simulink subsystem "User_Interface_Dashboard"  (R2024b)
settings: Solver=VariableStepAuto  StartTime=0.0  StopTime=10.0  RelTol=1e-3
undefined symbols (not defined in the file): NrLEDStrips, operatingMode, ts1ms, ts500us
libraries: SEPIC_utilities x6, simulink x1
settings Model: Creator=vlenzi  LastModifiedBy=vlenzi

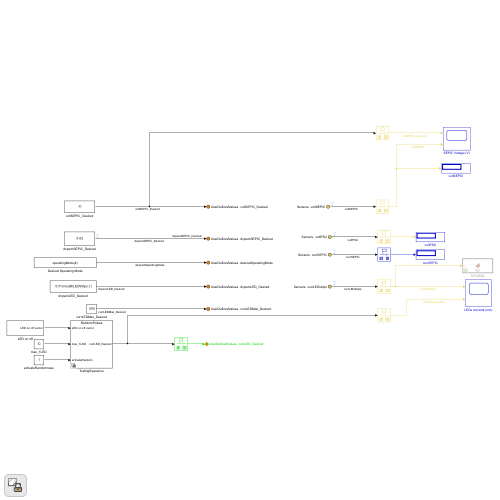
[thumbnail: Simulink's stored preview of the top-level diagram]
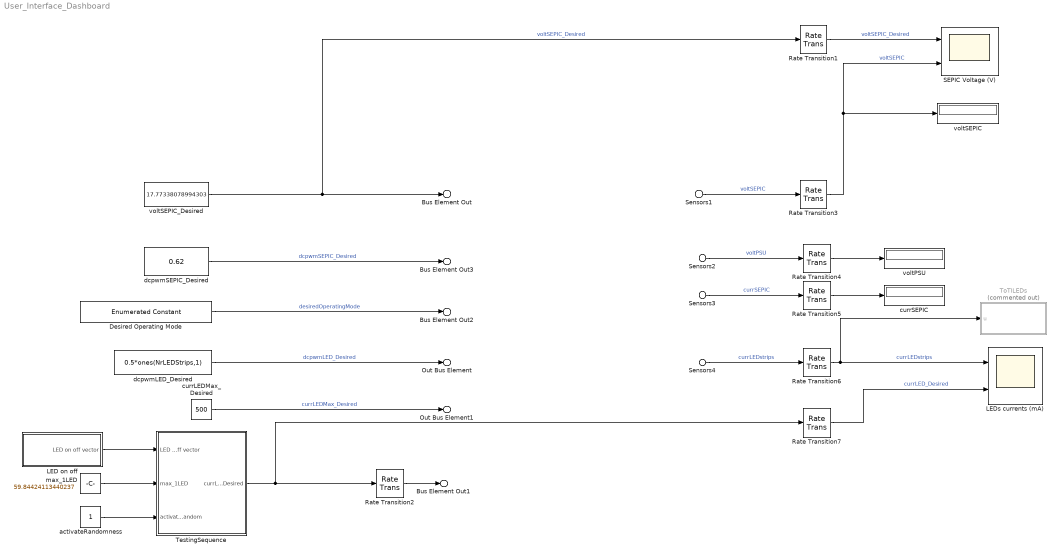
== system User_Interface_Dashboard ==
  Sensors1 : Inport  PortName=Sensors  Element=voltSEPIC
  Sensors3 : Inport  PortName=Sensors  Element=currSEPIC
  Sensors4 : Inport  PortName=Sensors  Element=currLEDstrips
  Sensors2 : Inport  PortName=Sensors  Element=voltPSU
  Desired Operating Mode : simulink/Sources/Enumerated Constant  OutDataTypeStr=Enum: operatingMode  Value=operatingMode(4)  SampleTime=-1
  LED on off : Subsystem
  LEDs currents (mA) : Scope  NumInputPorts=2
  Rate Transition{1,3..7} (6 alike) : RateTransition  Deterministic=off  OutPortSampleTime=ts10ms
  Rate Transition2 : RateTransition  Deterministic=off
  SEPIC Voltage (V) : Scope  NumInputPorts=2
  TestingSequence : Subsystem  Variant=on  VariantControlMode=label  VariantControl=Choice  LabelModeActiveChoice=Choice_1
  ToTILEDs : MATLAB Function  Commented=on  TreatAsAtomicUnit=on
  activateRandomness : Constant  OutDataTypeStr=single  SampleTime=-1
  currLEDMax_Desired : Constant  Value=500  OutDataTypeStr=single  SampleTime=-1
  currSEPIC : Display
  dcpwmLED_Desired : Constant  Value=0.5*ones(NrLEDStrips,1)  OutDataTypeStr=single  SampleTime=-1
  dcpwmSEPIC_Desired : Constant  Value=0.62  OutDataTypeStr=single  SampleTime=-1
  max_1LED : Constant  Value=59.84424113440237  OutDataTypeStr=single  SampleTime=-1
  voltPSU : Display
  voltSEPIC : Display
  voltSEPIC_Desired : Constant  Value=17.77338078994303  OutDataTypeStr=single  SampleTime=-1
  Bus Element Out1 : Outport  PortName=UserDefinedValues  Element=currLED_Desired
  Out Bus Element1 : Outport  PortName=UserDefinedValues  Element=currLEDMax_Desired
  Bus Element Out3 : Outport  PortName=UserDefinedValues  Element=dcpwmSEPIC_Desired
  Out Bus Element : Outport  PortName=UserDefinedValues  Element=dcpwmLED_Desired
  Bus Element Out2 : Outport  PortName=UserDefinedValues  Element=desiredOperatingMode
  Bus Element Out : Outport  PortName=UserDefinedValues  Element=voltSEPIC_Desired
  wires:
  voltSEPIC_Desired/1 -> Rate Transition1/1, Bus Element Out/1  "voltSEPIC_Desired"
  Desired Operating Mode/1 -> Bus Element Out2/1  "desiredOperatingMode"
  Sensors1/1 -> Rate Transition3/1  "voltSEPIC"
  Sensors2/1 -> Rate Transition4/1  "voltPSU"
  Sensors3/1 -> Rate Transition5/1  "currSEPIC"
  Sensors4/1 -> Rate Transition6/1  "currLEDstrips"
  dcpwmSEPIC_Desired/1 -> Bus Element Out3/1  "dcpwmSEPIC_Desired"
  dcpwmLED_Desired/1 -> Out Bus Element/1  "dcpwmLED_Desired"
  Rate Transition6/1 -> ToTILEDs/1(u), LEDs currents (mA)/1  "currLEDstrips"
  currLEDMax_Desired/1 -> Out Bus Element1/1  "currLEDMax_Desired"
  Rate Transition3/1 -> SEPIC Voltage (V)/2, voltSEPIC/1  "voltSEPIC"
  Rate Transition4/1 -> voltPSU/1
  Rate Transition5/1 -> currSEPIC/1
  Rate Transition1/1 -> SEPIC Voltage (V)/1  "voltSEPIC_Desired"
  TestingSequence/1(currLED_Desired) -> Rate Transition7/1, Rate Transition2/1
  Rate Transition7/1 -> LEDs currents (mA)/2  "currLED_Desired"
  max_1LED/1 -> TestingSequence/2(max_1LED)
  LED on off/1(LED on off vector) -> TestingSequence/1(LED on off vector)
  activateRandomness/1 -> TestingSequence/3(activateRandom)
  Rate Transition2/1 -> Bus Element Out1/1

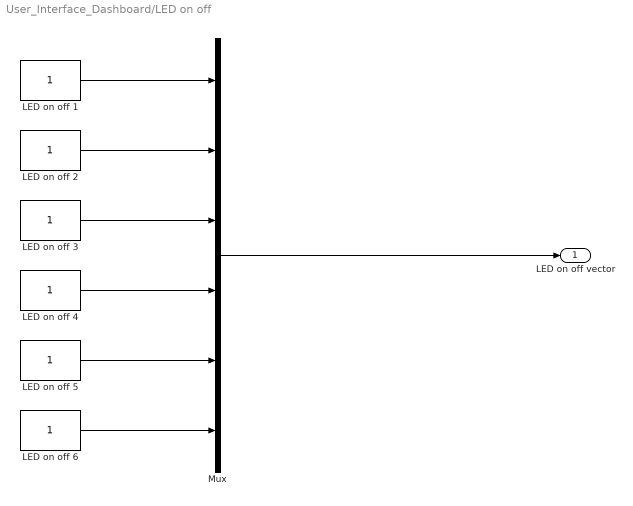
== system User_Interface_Dashboard/LED on off ==
  LED on off {1..6} (6 alike) : Constant  OutDataTypeStr=single  SampleTime=-1
  Mux : Mux  Inputs=6
  LED on off vector : Outport
  wires:
  LED on off 3/1 -> Mux/3
  LED on off 5/1 -> Mux/5
  LED on off 1/1 -> Mux/1
  LED on off 4/1 -> Mux/4
  LED on off 2/1 -> Mux/2
  LED on off 6/1 -> Mux/6
  Mux/1 -> LED on off vector/1

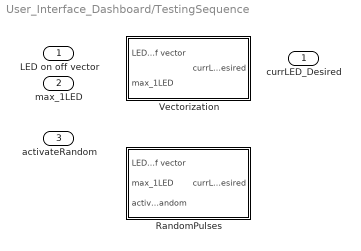
== system User_Interface_Dashboard/TestingSequence ==
  LED on off vector : Inport
  max_1LED : Inport  Port=2
  activateRandom : Inport  Port=3
  RandomPulses : Subsystem  VariantControl=Choice_1
  Vectorization : Subsystem  VariantControl=Choice
  currLED_Desired : Outport

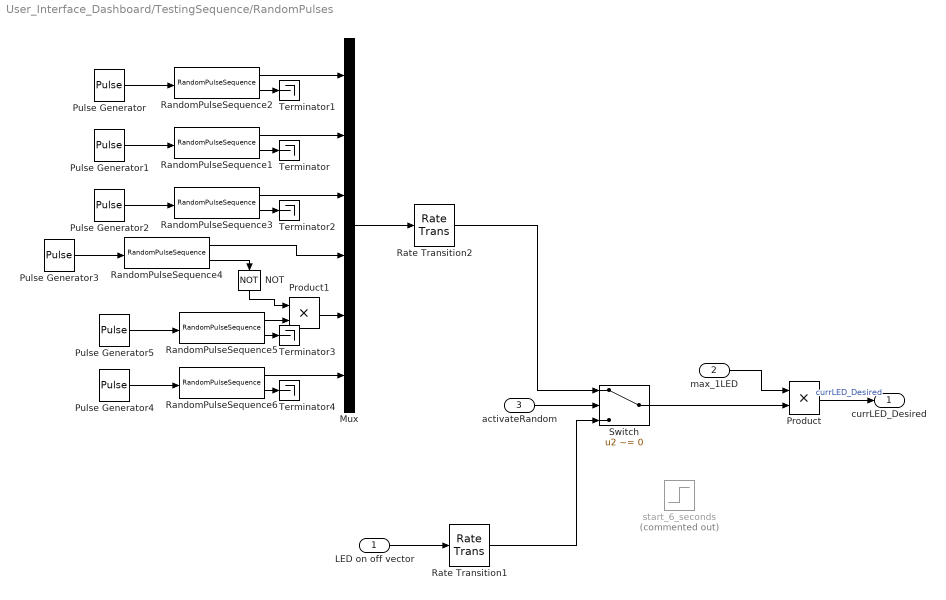
== system User_Interface_Dashboard/TestingSequence/RandomPulses ==
  LED on off vector : Inport
  max_1LED : Inport  Port=2
  activateRandom : Inport  Port=3
  Mux : Mux  Inputs=6
  NOT : Logic  Operator=NOT  AllPortsSameDT=off  OutDataTypeStr=boolean
  Product : Product  OutDataTypeStr=single
  Product1 : Product
  Pulse Generator : DiscretePulseGenerator  Period=2*(1/ts500us)  PulseWidth=1*(1/ts500us)  SampleTime=ts500us
  Pulse Generator1 : DiscretePulseGenerator  Period=2*(1/ts500us)  PulseWidth=1*(1/ts500us)  PhaseDelay=1*400  SampleTime=ts500us
  Pulse Generator2 : DiscretePulseGenerator  Period=2*(1/ts500us)  PulseWidth=1*(1/ts500us)  PhaseDelay=2*400  SampleTime=ts500us
  Pulse Generator3 : DiscretePulseGenerator  Period=2*(1/ts500us)  PulseWidth=1*(1/ts500us)  PhaseDelay=3*400  SampleTime=ts500us
  Pulse Generator4 : DiscretePulseGenerator  Period=2*(1/ts500us)  PulseWidth=1*(1/ts500us)  PhaseDelay=5*400  SampleTime=ts500us
  Pulse Generator5 : DiscretePulseGenerator  Period=2*(1/ts500us)  PulseWidth=1*(1/ts500us)  PhaseDelay=4*400  SampleTime=ts500us
  RandomPulseSequence1 : SEPIC_utilities/RandomPulseSequence  seed=2  sampleTime=4
  RandomPulseSequence2 : SEPIC_utilities/RandomPulseSequence  seed=1  sampleTime=4
  RandomPulseSequence3 : SEPIC_utilities/RandomPulseSequence  seed=3  sampleTime=4
  RandomPulseSequence4 : SEPIC_utilities/RandomPulseSequence  seed=4  sampleTime=4
  RandomPulseSequence5 : SEPIC_utilities/RandomPulseSequence  seed=5  sampleTime=4
  RandomPulseSequence6 : SEPIC_utilities/RandomPulseSequence  seed=6  sampleTime=4
  Rate Transition1 : RateTransition  Deterministic=off
  Rate Transition2 : RateTransition  Deterministic=off
  Switch : Switch  Criteria=u2 ~= 0  SaturateOnIntegerOverflow=off  InputSameDT=off
  Terminator{,1..4} (5 alike) : Terminator
  start_6_seconds : Step  Commented=on  Time=6  SampleTime=ts1ms
  currLED_Desired : Outport
  wires:
  Rate Transition1/1 -> Switch/3
  Rate Transition2/1 -> Switch/1
  LED on off vector/1 -> Rate Transition1/1
  Switch/1 -> Product/2
  activateRandom/1 -> Switch/2
  max_1LED/1 -> Product/1
  Product/1 -> currLED_Desired/1  "currLED_Desired"
  RandomPulseSequence3/2 -> Terminator2/1
  RandomPulseSequence2/1 -> Mux/1
  RandomPulseSequence5/1 -> Product1/2
  Pulse Generator4/1 -> RandomPulseSequence6/1
  Mux/1 -> Rate Transition2/1
  Pulse Generator5/1 -> RandomPulseSequence5/1
  Pulse Generator1/1 -> RandomPulseSequence1/1
  NOT/1 -> Product1/1
  RandomPulseSequence1/2 -> Terminator/1
  RandomPulseSequence4/2 -> NOT/1
  RandomPulseSequence3/1 -> Mux/3
  RandomPulseSequence4/1 -> Mux/4
  Pulse Generator2/1 -> RandomPulseSequence3/1
  Product1/1 -> Mux/5
  RandomPulseSequence1/1 -> Mux/2
  Pulse Generator/1 -> RandomPulseSequence2/1
  Pulse Generator3/1 -> RandomPulseSequence4/1
  RandomPulseSequence2/2 -> Terminator1/1
  RandomPulseSequence6/1 -> Mux/6
  RandomPulseSequence6/2 -> Terminator4/1
  RandomPulseSequence5/2 -> Terminator3/1

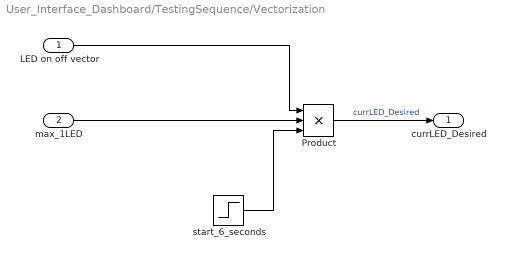
== system User_Interface_Dashboard/TestingSequence/Vectorization ==
  LED on off vector : Inport
  max_1LED : Inport  Port=2
  Product : Product  Inputs=3  OutDataTypeStr=single
  start_6_seconds : Step  Time=6  SampleTime=ts1ms
  currLED_Desired : Outport
  wires:
  LED on off vector/1 -> Product/1
  max_1LED/1 -> Product/2
  Product/1 -> currLED_Desired/1  "currLED_Desired"
  start_6_seconds/1 -> Product/3

== matlab function User_Interface_Dashboard/ToTILEDs ==
  data: u input
function fcn(u)
%%%%%%%%%%%%%%%%%%%%%%%%%%%%%%%%%%%%%%%%%%%%%%%%%%%%%%%%%%%%%%%%%%%%%%%%%%%%%%%%
% Function: fcn()
% Goal    : Write new values to the groups of LEDs
% IN      : - u : vector of new values for each LEDs groups
% IN/OUT  : -
% OUT     : -
%%%%%%%%%%%%%%%%%%%%%%%%%%%%%%%%%%%%%%%%%%%%%%%%%%%%%%%%%%%%%%%%%%%%%%%%%%%%%%%%
  coder.extrinsic('evalin');
  appObj = evalin('base','objLEDs');
  funObj = 'setTiLeds';
  % Write new values to each LEDs group
  for n=1:1:length(u)
    feval(funObj,appObj,u(n),n);
  end
end
